simulink model "usrp_fm_mono"  (R2014b)
settings: Solver=ode45  StartTime=0.0  StopTime=inf  RelTol=1e-3
PreLoadFcn:
  | %%%%%%%%%%%%%%%%%%%%%%%%%%%%%%%%%%%%%%%%%%%%%%%%%%%%%%%%%%%%%%%%%%%%%%%%%%%
  | % check to see if Simulink library folder is missing from the MATLAB path %
  | %%%%%%%%%%%%%%%%%%%%%%%%%%%%%%%%%%%%%%%%%%%%%%%%%%%%%%%%%%%%%%%%%%%%%%%%%%%
  | if isempty(strfind(path, 'rtlsdr_book_library'))
  | 
  |     % create error window
  |     fig_error = figure(...
  |         'Name', 'Error: RTL-SDR Book Library',...
  |         'Toolbar','none',...
  |         'MenuBar','none',...
  |         'NumberTitle','off',...
  |         'Resize','off',...
  |         'WindowStyle','modal');
  |     fig_error.Position(3) = 600;
  |     fig_error.Position(4) = 150;
  |     fig_axes = axes(...
  |         'Parent',fig_error,...
  |         'Position',[0,0,1,1],...
  |         'visible','off');
  |     % error message
  |     t_title = text(.05,.8,...
  |         'MISSING DIRECTORIES',...
  |         'FontSize',11.5);
  |     t_body = text(.075,.6,...
  |         [{'Simulink cannot find the  \it{<root>}\rm / \it{rtlsdr\_book\_library}\rm  folder in the \it{MATLAB Path}\rm.'},...
  |         {'Please set the MATLAB path following the instructions given in Exercise 2.4.'}],...
  |         'FontSize',10.5);
  |     % buttons
  |     btn_path = uicontrol(...
  |         'Parent',fig_error,...
  |         'String','Set Path Now',...
  |         'FontSize',10,...
  |         'Callback', 'pathtool; close(fig_error);',...
  |         'Position', [fig_error.Position(3)/2-210, 30, 200, 30]);
  |     btn_abort = uicontrol(...
  |         'Parent',fig_error,...
  |         'String','No thanks',...
  |         'FontSize',10,...
  |         'Callback', 'close(fig_error); abort=1;',...
  |         'Position', [fig_error.Position(3)/2+10, 30, 200, 30]);
  | 
  |     % pause to allow user to interact with error box
  |     uiwait(fig_error);
  | 
  |     % abort simulation
  |     try
  |         if abort==1
  |             set_param(gcs, 'SimulationCommand', 'stop');
  |         end
  |     end
  | 
  |     % if user has set path, allow diagram to be updated
  |     if ~exist('abort','var')
  |         % create error window
  |         fig_update = figure(...
  |             'Name', 'Update Diagram',...
  |             'Toolbar','none',...
  |             'MenuBar','none',...
  |             'NumberTitle','off',...
  |             'Resize','off');
  |         fig_update.Position(3) = 400;
  |         fig_update.Position(4) = 120;
  |         fig_axes = axes(...
  |             'Parent',fig_update,...
  |             'Position',[0,0,1,1],...
  |             'visible','off');
  |         % instruction message
  |         t_body = text(.075,.7,...
  |             'Once you have set the path, update the block diagram',...
  |             'FontSize',10.5);
  |         % button
  |         btn_update = uicontrol(...
  |             'Parent',fig_update,...
  |             'String','Update Block Diagram',...
  |             'FontSize',10,...
  |             'Callback', 'set_param(gcs,''SimulationCommand'',''update''); close(gcf)',...
  |             'Position', [fig_update.Position(3)/2-100, 30, 200, 30]);
  |     end
  | 
  |     % clear error components
  |     clear('fig_error','fig_update','fig_axes','t_title','t_body','btn_path','btn_abort','btn_update','abort');
  | 
  | end
  | %%%%%%%%%%%%%%%%%%%%%%%%%%%%%%%%%%%%%%%%%%%%%%%%%%%%%%%%%%%%%%%%%%%%%%%%%%%
undefined symbols (not defined in the file): fdesignblkfcn, gcbh, startfcn_spectrum_analyzer
libraries: dspmlti4 x3, dspvision x1, rtlsdr_book_library x1, commsdrhw_v2 x1
CloseFcn:
  | closefcn_model
Description:
  | Software, Simulation Examples and Design Exercises Licence Agreement
  | 
  | This license agreement refers to the simulation examples, design exercises and files,
  | and associated software MATLAB and Simulink resources that accompany the book:
  | 
  |      Title: Software Defined Radio using MATLAB & Simulink and the RTL-SDR
  |      Published by Strathclyde Academic Media, 2015
  |      Authored by Robert W. Stewart, Kenneth W. Barlee, Dale S.W. Atkinson,
  |      and Louise H. Crockett
  | 
  | and made available as a download from, www.desktopSDR.com or variously acquired
  | by other means such as via USB storage, cloud storage, disk or any other electronic
  | or optical or magnetic storage mechanism. These files and associated software may
  | be used subject to the terms of agreement of the conditions below:
  | 
  |     Copyright © 2015 Robert W. Stewart, Kenneth W. Barlee, Dale S.W. Atkinson,
  |     and Louise H. Crockett
  |     All rights reserved.
  | 
  | Redistribution and use in source and binary forms, with or without modification, are
  | permitted provided that the following conditions are met:
  | 
  |    1.  Redistributions of source code must retain the above copyright notice, this list of
  |         conditions and the following disclaimer.
  | 
  |    2.  Redistributions in binary form must reproduce the above copyright notice, this
  |         list of conditions and the following disclaimer in the documentation and/or other
  |         materials provided with the distribution.
  | 
  |    3.  Neither the name of the copyright holder nor the names of its contributors may
  |         be used to endorse or promote products derived from this software without
  |         specific prior written permission.
  | 
  |    4.  In all cases, the software is, and all modifications and derivatives of the
  |         software shall be, licensed to you solely for use in conjunction with The
  |         MathWorks, Inc. products and service offerings.
  | 
  | THIS SOFTWARE IS PROVIDED BY THE COPYRIGHT HOLDERS AND CONTRIBUTORS
  | "AS IS" AND ANY EXPRESS OR IMPLIED WARRANTIES, INCLUDING, BUT NOT LIMITED
  | TO, THE IMPLIED WARRANTIES OF MERCHANTABILITY AND FITNESS FOR A
  | PARTICULAR PURPOSE ARE DISCLAIMED. IN NO EVENT SHALL THE COPYRIGHT
  | HOLDER OR CONTRIBUTORS BE LIABLE FOR ANY DIRECT, INDIRECT, INCIDENTAL,
  | SPECIAL, EXEMPLARY, OR CONSEQUENTIAL DAMAGES (INCLUDING, BUT NOT
  | LIMITED TO, PROCUREMENT OF SUBSTITUTE GOODS OR SERVICES; LOSS OF USE,
  | DATA, OR PROFITS; OR BUSINESS INTERRUPTION) HOWEVER CAUSED AND ON ANY
  | THEORY OF LIABILITY, WHETHER IN CONTRACT, STRICT LIABILITY, OR TORT
  | (INCLUDING NEGLIGENCE OR OTHERWISE) ARISING IN ANY WAY OUT OF THE USE
  | OF THIS SOFTWARE, EVEN IF ADVISED OF THE POSSIBILITY OF SUCH DAMAGE.
  | 
  | 
  | Audio Tracks used in Simulations Examples and Design Exercises
  | 
  | The music and vocal files used within the Examples files and software within the book
  | were variously written, arranged, performed, recorded and produced by Garrey Rice,
  | Adam Struth, Jamie Struth, Iain Thistlethwaite and also Marshall Craigmyle who
  | collectively, and individually where appropriate, assert and retain all of their copyright,
  | performance and artistic rights. Permission to use and reproduce this music is
  | granted for all purposes associated with MATLAB and Simulink software and the
  | simulation examples and design exercises files that accompany this book. Requests to
  | use the music for any other purpose should be directed to: info@desktopSDR.com.
  | For information on music track names, full credits, and links to the musicians please
  | refer to www.desktopSDR.com/more/audio.
settings Model: SimulationMode=accelerator  Creator=desktopSDR Team  LastModifiedBy=desktopSDR Team
settings DataIOCC: LimitDataPoints=off  SaveOutput=off  SignalLogging=off  SaveTime=off

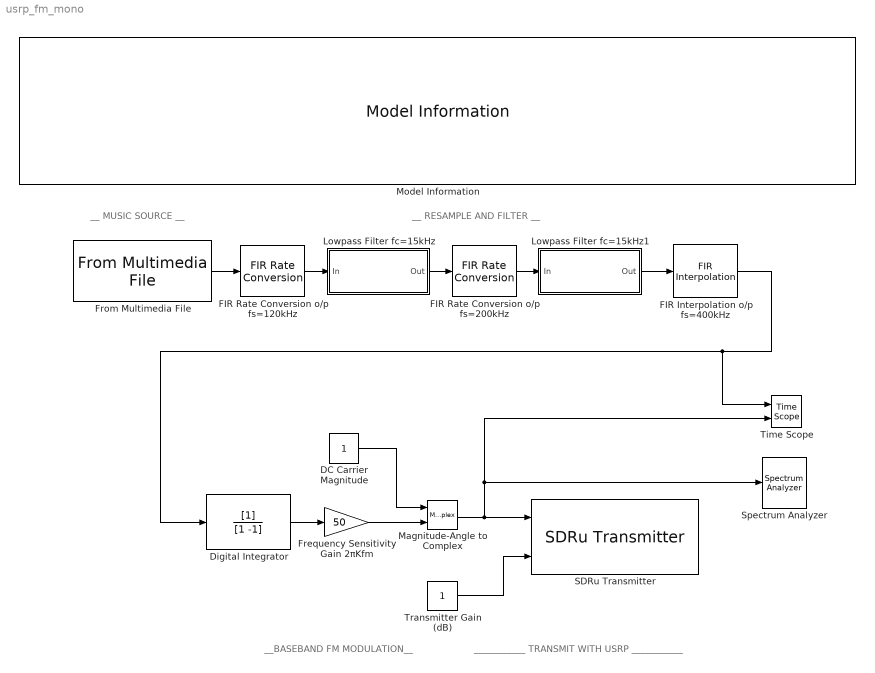
== system usrp_fm_mono ==
  note: __ MUSIC SOURCE __
  note: __ RESAMPLE AND FILTER __
  note: ___________ TRANSMIT WITH USRP ___________
  note: __BASEBAND FM MODULATION__
  DC Carrier Magnitude : Constant
  Digital Integrator : DiscreteFilter  Denominator=[1 -1]  InputProcessing=Columns as channels (frame based)  FilterStructure=Direct form II transposed  a0EqualsOne=on
  FIR Interpolation o/p fs=400kHz : dspmlti4/FIR Interpolation  h=firpm(100, [0 15e3 30e3 400e3/2]/(400e3/2), [1 1 0 0], [1 1],20)  L=2  framing=Allow multirate processing  outputBufInitCond=0  InputProcessing=Columns as channels (frame based)  firstCoeffDataTypeStr=Inherit: Same word length as input  firstCoeffLastDataTypeStr=Inherit: Same word length as input  firstCoeffMin=[]  firstCoeffMax=[]  outputDataTypeStr=Inherit: Same as accumulator  outputLastDataTypeStr=Inherit: Same as accumulator  outputMin=[]  outputMax=[]  roundingMode=Floor  overflowMode=off  FilterSource=Specify via dialog  FilterObject=Hm_firinterp
  FIR Rate Conversion o/p fs=120kHz : dspmlti4/FIR Rate Conversion  L=5  h=firpm(50, [0 15e3 24e3 240e3/2]/(240e3/2), [1 1 0 0], [1 1],20)  M=2  firstCoeffDataTypeStr=Inherit: Same word length as input  firstCoeffLastDataTypeStr=Inherit: Same word length as input  firstCoeffMin=[]  firstCoeffMax=[]  outputDataTypeStr=Inherit: Same as accumulator  outputLastDataTypeStr=Inherit: Same as accumulator  outputMin=[]  outputMax=[]  roundingMode=Floor  overflowMode=off  FilterSource=Specify via dialog  FilterObject=Hm_firsrc
  FIR Rate Conversion o/p fs=200kHz : dspmlti4/FIR Rate Conversion  L=5  h=firpm(100, [0 15e3 30e3 600e3/2]/(600e3/2), [1 1 0 0], [1 1],20)  M=3  firstCoeffDataTypeStr=Inherit: Same word length as input  firstCoeffLastDataTypeStr=Inherit: Same word length as input  firstCoeffMin=[]  firstCoeffMax=[]  outputDataTypeStr=Inherit: Same as accumulator  outputLastDataTypeStr=Inherit: Same as accumulator  outputMin=[]  outputMax=[]  roundingMode=Floor  overflowMode=off  FilterSource=Specify via dialog  FilterObject=Hm_firsrc
  Frequency Sensitivity Gain 2πKfm : Gain  Gain=50
  From Multimedia File : dspvision/From Multimedia File  inputFilename=../../audio_sources/music5_mono48kHz.wav  loop=on  numPlays=inf  outputStreams=Audio only  videoDataType=single  audioDataType=double  inheritSampleTime=on  userDefinedSampleTime=1/30  noAudioOutput=off  isIntensityVideo=off  fourcc=RGB  colorVideoFormat=One multidimensional signal  outputEOF=off  dataOrg=Column-major  audioFrameSize=600  computeAudioFrameSize=off  outSamplingMode=Sample based
  Lowpass Filter fc=15kHz : Subsystem  DialogController=fdesignblkfcn  InitFcn=fdesignblkfcn(gcbh, {'InitFcn'});  mask(Lowpass Filter){}
      mask help: Design a lowpass filter
      settings: CopyFcn=fdesignblkfcn(gcbh, {'CopyFcn'});
      mask Help: helpview(mapfilelocation('dsp'), 'dsplowpassfilter');
      mask Display: disp('Lowpass')
  Lowpass Filter fc=15kHz1 : Subsystem  DialogController=fdesignblkfcn  InitFcn=fdesignblkfcn(gcbh, {'InitFcn'});  mask(Lowpass Filter){}
      mask help: Design a lowpass filter
      settings: CopyFcn=fdesignblkfcn(gcbh, {'CopyFcn'});
      mask Help: helpview(mapfilelocation('dsp'), 'dsplowpassfilter');
      mask Display: disp('Lowpass')
  Magnitude-Angle to Complex : MagnitudeAngleToComplex
  Model Information : rtlsdr_book_library/Additional Tools/Model Information/Model Information
  SDRu Transmitter : commsdrhw_v2/SDRu Transmitter  rxtx=tx  platform=N200/N210/USRP2  USRP2_IP='169.254.10.2'  USRP_IP_X300='192.168.10.2'  USRP_IP_X310='192.168.10.2'  USRP_serialNumB200=''  USRP_serialNumB210=''  centerFrequency=433.9e6  centerFrequencySrc=Dialog  loOffset=250e3  loOffsetSrc=Dialog  masterClkRateB200=32e6  masterClkRateB210=32e6  masterClkRateX300=200e6  masterClkRateX310=200e6  masterClkRateParam=100e6  gain=10  gainSrc=Input port  decimInterp=250  decimInterpSrc=Dialog  USRP2_IP_NUM=[49 54 57 46 50 53 52 46 49 48 46 50]  frameLength=362  outputDatatype=int16  overrunUnderrunPort=off  sampleTime=1  dboardInfo=|  HOST_DATA_PORT=30000  HOST_CONTROL_PORT=30001  USRP2_DATA_PORT=32769  USRP2_CONTROL_PORT=32768  bufferMode=Continuous streaming  EnableBurstMode=off  NumFramesInBurst=100  USRP_ID='169.254.10.2'
      | dbid: 0
      |           dbName: 'no db found'
      |          freqMin: 0
      |          freqMax: 0
      |          gainMin: 0
      |          gainMax: 0
      |     gainStepSize: 0
  Spectrum Analyzer : SpectrumAnalyzer  StartFcn=startfcn_spectrum_analyzer;
  Time Scope : TimeScope  StartFcn=startfcn_time_scope  DefaultConfigurationName=spbscopes.TimeScopeBlockCfg  NumInputPorts=2
  Transmitter Gain (dB) : Constant
  wires:
  Digital Integrator/1 -> Frequency Sensitivity Gain 2πKfm/1
  DC Carrier Magnitude/1 -> Magnitude-Angle to Complex/1
  Frequency Sensitivity Gain 2πKfm/1 -> Magnitude-Angle to Complex/2
  FIR Rate Conversion o/p fs=120kHz/1 -> Lowpass Filter fc=15kHz/1(In)
  FIR Rate Conversion o/p fs=200kHz/1 -> Lowpass Filter fc=15kHz1/1(In)
  Lowpass Filter fc=15kHz/1(Out) -> FIR Rate Conversion o/p fs=200kHz/1
  Lowpass Filter fc=15kHz1/1(Out) -> FIR Interpolation o/p fs=400kHz/1
  From Multimedia File/1 -> FIR Rate Conversion o/p fs=120kHz/1
  Magnitude-Angle to Complex/1 -> Time Scope/2, Spectrum Analyzer/1, SDRu Transmitter/1
  Transmitter Gain (dB)/1 -> SDRu Transmitter/2
  FIR Interpolation o/p fs=400kHz/1 -> Time Scope/1, Digital Integrator/1

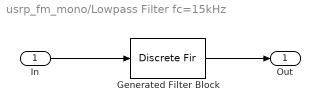
== system usrp_fm_mono/Lowpass Filter fc=15kHz ==
  In : Inport
  Generated Filter Block : DiscreteFir  Tag=BlockMethodSubSystem  Coefficients=[1.0066150157102917e-06 -3.2372912431162512e-07 -4.2855970962183648e-06 -6.4851915295408206e-06 1.1717483061228179e-06 1.7999936427846823e-05 2.493046729014389e-05 -1.4808943362511689e-06 -5.3046338186012682e-05 -7.3197278794272686e-05 -3.7341877515233612e-06 0.00012742290534606515 0.00018107701577170057 2.7076661862873555e-05 -0.00026580210462364947 -0.00039594194262893343 -9.4448464465583156e-05 0.00049781587168696727 0.00078691512979048826 0.00025206984549170633 -0.00085415830032188438 -0.0014480215906730409 -0.0005745982846593774 0.0013606253311563695 0.0025005155900828099 0.0011744236731699614 -0.0020309057051019633 -0.0040963730097355626 -0.0022137908753939485 0.0028595729058621838 0.0064285354446839563 0.0039255782564997519 -0.0038170716802022513 -0.0097615391999868861 -0.0066593808949039213 0.0048484130870308489 0.01451763771418605 0.011001298720289977 -0.005876687193845054 -0.021525527264800982 -0.018130512861211721 0.0068114950814328916 0.032852156569452853 0.031128500274350789 -0.0075612028480277179 -0.055644906262703783 -0.062236096788139586 0.0080468647939795461 0.1405226341844866 0.27087416189070773 0.32511828328973702 0.27087416189070773 0.1405226341844866 0.0080468647939795461 -0.062236096788139586 -0.055644906262703783 -0.0075612028480277179 0.031128500274350789 0.032852156569452853 0.0068114950814328916 -0.018130512861211721 -0.021525527264800982 -0.005876687193845054 0.011001298720289977 0.01451763771418605 0.0048484130870308489 -0.0066593808949039213 -0.0097615391999868861 -0.0038170716802022513 0.0039255782564997519 0.0064285354446839563 0.0028595729058621838 -0.0022137908753939485 -0.0040963730097355626 -0.0020309057051019633 0.0011744236731699614 0.0025005155900828099 0.0013606253311563695 -0.0005745982846593774 -0.0014480215906730409 -0.00085415830032188438 0.00025206984549170633 0.00078691512979048826 0.00049781587168696727 -9.4448464465583156e-05 -0.00039594194262893343 -0.00026580210462364947 2.7076661862873555e-05 0.00018107701577170057 0.00012742290534606515 -3.7341877515233612e-06 -7.3197278794272686e-05 -5.3046338186012682e-05 -1.4808943362511689e-06 2.493046729014389e-05 1.7999936427846823e-05 1.1717483061228179e-06 -6.4851915295408206e-06 -4.2855970962183648e-06 -3.2372912431162512e-07 1.0066150157102917e-06]  InputProcessing=Columns as channels (frame based)
  Out : Outport
  wires:
  In/1 -> Generated Filter Block/1
  Generated Filter Block/1 -> Out/1

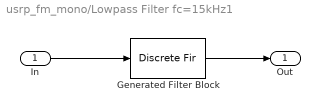
== system usrp_fm_mono/Lowpass Filter fc=15kHz1 ==
  In : Inport
  Generated Filter Block : DiscreteFir  Tag=BlockMethodSubSystem  Coefficients=[-3.9862720454903627e-05 -0.00014657359993843635 -0.00011759560799873501 -9.4259669875135837e-05 2.8852610450880716e-05 0.0001984781413238418 0.00036033219713356418 0.00042009143322916629 0.0003003690856970864 -1.8880541914720467e-05 -0.00046390987396872961 -0.00086938985440667446 -0.0010266965394373679 -0.00077121296820129763 -7.7045410617431704e-05 0.00088478263028423439 0.0017640753835437427 0.0021395062069204862 0.0016915286561505316 0.00037795269460455473 -0.0014697766813936161 -0.00319272956394914 -0.0040112545771060684 -0.0033370382579112497 -0.0010792693451485813 0.0021937899502219556 0.0053412798832452417 0.0070040521498317175 0.0061335387718721868 0.0025064760763200905 -0.0029953437256820563 -0.0085088088823360337 -0.011748614384222341 -0.01085970914530522 -0.0052730845193915826 0.0037829510317805323 0.013387688210584852 0.019728260160446341 0.019416518586779744 0.010913709644639447 -0.0044503446832664419 -0.022307450519016538 -0.036128161698530982 -0.038995227023162361 -0.025789046562521671 0.0048982160773998083 0.049780052164918327 0.10123304856297781 0.14899378235251026 0.18275965613792694 0.19494397685370951 0.18275965613792694 0.14899378235251026 0.10123304856297781 0.049780052164918327 0.0048982160773998083 -0.025789046562521671 -0.038995227023162361 -0.036128161698530982 -0.022307450519016538 -0.0044503446832664419 0.010913709644639447 0.019416518586779744 0.019728260160446341 0.013387688210584852 0.0037829510317805323 -0.0052730845193915826 -0.01085970914530522 -0.011748614384222341 -0.0085088088823360337 -0.0029953437256820563 0.0025064760763200905 0.0061335387718721868 0.0070040521498317175 0.0053412798832452417 0.0021937899502219556 -0.0010792693451485813 -0.0033370382579112497 -0.0040112545771060684 -0.00319272956394914 -0.0014697766813936161 0.00037795269460455473 0.0016915286561505316 0.0021395062069204862 0.0017640753835437427 0.00088478263028423439 -7.7045410617431704e-05 -0.00077121296820129763 -0.0010266965394373679 -0.00086938985440667446 -0.00046390987396872961 -1.8880541914720467e-05 0.0003003690856970864 0.00042009143322916629 0.00036033219713356418 0.0001984781413238418 2.8852610450880716e-05 -9.4259669875135837e-05 -0.00011759560799873501 -0.00014657359993843635 -3.9862720454903627e-05]  InputProcessing=Columns as channels (frame based)
  Out : Outport
  wires:
  Generated Filter Block/1 -> Out/1
  In/1 -> Generated Filter Block/1
